simulink model "CL1CM2"  (R2024b)
settings: Solver=VariableStepAuto  StartTime=0.0  StopTime=10.0  RelTol=1e-3
settings Model: Creator=jeonghyun  LastModifiedBy=gluts

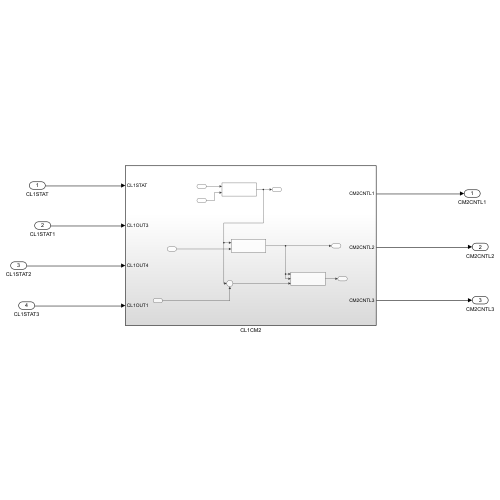
[thumbnail: Simulink's stored preview of the top-level diagram]
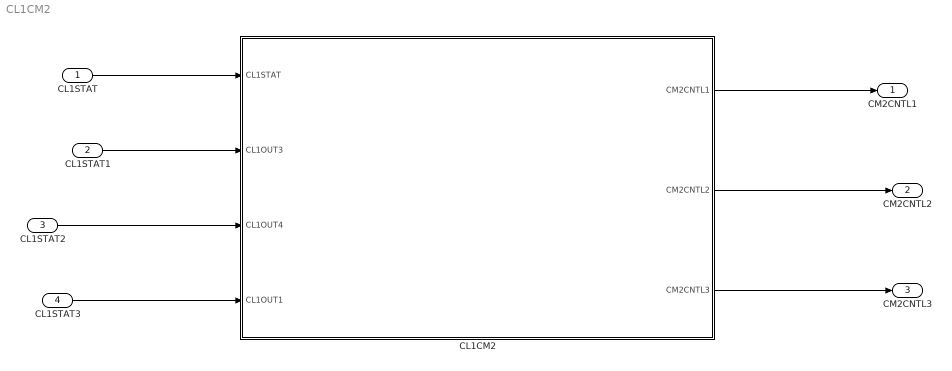
== system CL1CM2 ==
  CL1STAT : Inport
  CL1STAT1 : Inport  Port=2
  CL1STAT2 : Inport  Port=3
  CL1STAT3 : Inport  Port=4
  CL1CM2 : Subsystem
  CM2CNTL1 : Outport
  CM2CNTL2 : Outport  Port=2
  CM2CNTL3 : Outport  Port=3
  wires:
  CL1STAT/1 -> CL1CM2/1(CL1STAT)
  CL1STAT1/1 -> CL1CM2/2(CL1OUT3)
  CL1STAT2/1 -> CL1CM2/3(CL1OUT4)
  CL1STAT3/1 -> CL1CM2/4(CL1OUT1)
  CL1CM2/1(CM2CNTL1) -> CM2CNTL1/1
  CL1CM2/2(CM2CNTL2) -> CM2CNTL2/1
  CL1CM2/3(CM2CNTL3) -> CM2CNTL3/1

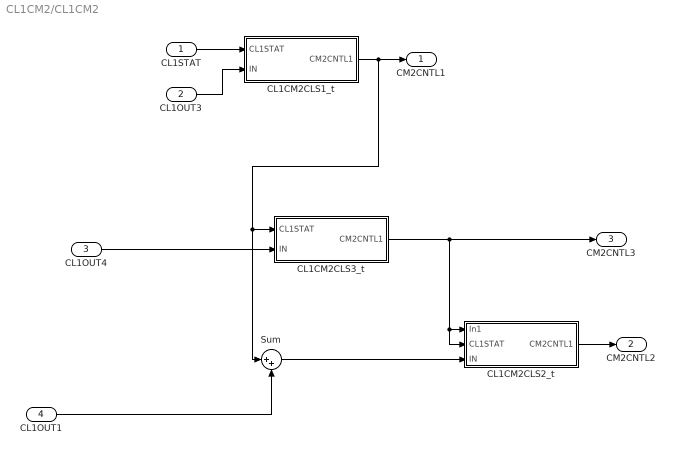
== system CL1CM2/CL1CM2 ==
  CL1STAT : Inport
  CL1OUT3 : Inport  Port=2
  CL1OUT4 : Inport  Port=3
  CL1OUT1 : Inport  Port=4
  CL1CM2CLS1_t : Subsystem
  CL1CM2CLS2_t : Subsystem
  CL1CM2CLS3_t : Subsystem
  Sum : Sum  Inputs=|++
  CM2CNTL1 : Outport
  CM2CNTL2 : Outport  Port=2
  CM2CNTL3 : Outport  Port=3
  wires:
  CL1STAT/1 -> CL1CM2CLS1_t/1(CL1STAT)
  CL1CM2CLS2_t/1(CM2CNTL1) -> CM2CNTL2/1
  CL1OUT3/1 -> CL1CM2CLS1_t/2(IN)
  CL1CM2CLS1_t/1(CM2CNTL1) -> CM2CNTL1/1, Sum/1, CL1CM2CLS3_t/1(CL1STAT)
  CL1OUT4/1 -> CL1CM2CLS3_t/2(IN)
  CL1CM2CLS3_t/1(CM2CNTL1) -> CL1CM2CLS2_t/1(In1), CL1CM2CLS2_t/2(CL1STAT), CM2CNTL3/1
  CL1OUT1/1 -> Sum/2
  Sum/1 -> CL1CM2CLS2_t/3(IN)

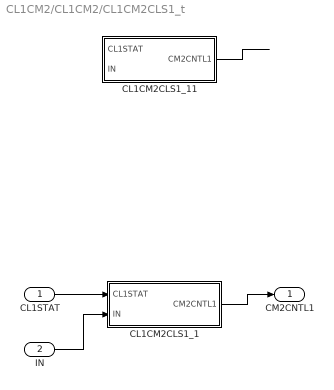
== system CL1CM2/CL1CM2/CL1CM2CLS1_t ==
  CL1STAT : Inport
  IN : Inport  Port=2
  CL1CM2CLS1_1 : Subsystem
  CL1CM2CLS1_11 : Subsystem
  CM2CNTL1 : Outport
  wires:
  CL1STAT/1 -> CL1CM2CLS1_1/1(CL1STAT)
  IN/1 -> CL1CM2CLS1_1/2(IN)
  CL1CM2CLS1_1/1(CM2CNTL1) -> CM2CNTL1/1
  CL1CM2CLS1_11/1(CM2CNTL1) -> ?
  ? -> CL1CM2CLS1_11/1(CL1STAT)
  ? -> CL1CM2CLS1_11/2(IN)

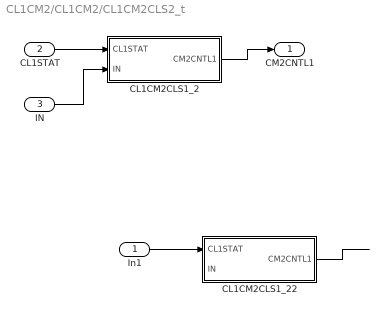
== system CL1CM2/CL1CM2/CL1CM2CLS2_t ==
  In1 : Inport
  CL1STAT : Inport  Port=2
  IN : Inport  Port=3
  CL1CM2CLS1_2 : Subsystem
  CL1CM2CLS1_22 : Subsystem
  CM2CNTL1 : Outport
  wires:
  CL1STAT/1 -> CL1CM2CLS1_2/1(CL1STAT)
  CL1CM2CLS1_2/1(CM2CNTL1) -> CM2CNTL1/1
  IN/1 -> CL1CM2CLS1_2/2(IN)
  In1/1 -> CL1CM2CLS1_22/1(CL1STAT)
  CL1CM2CLS1_22/1(CM2CNTL1) -> ?
  ? -> CL1CM2CLS1_22/2(IN)

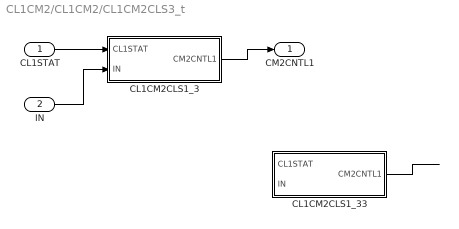
== system CL1CM2/CL1CM2/CL1CM2CLS3_t ==
  CL1STAT : Inport
  IN : Inport  Port=2
  CL1CM2CLS1_3 : Subsystem
  CL1CM2CLS1_33 : Subsystem
  CM2CNTL1 : Outport
  wires:
  CL1CM2CLS1_3/1(CM2CNTL1) -> CM2CNTL1/1
  CL1STAT/1 -> CL1CM2CLS1_3/1(CL1STAT)
  IN/1 -> CL1CM2CLS1_3/2(IN)
  ? -> CL1CM2CLS1_33/1(CL1STAT)
  CL1CM2CLS1_33/1(CM2CNTL1) -> ?
  ? -> CL1CM2CLS1_33/2(IN)

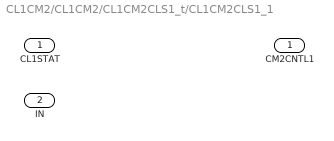
== system CL1CM2/CL1CM2/CL1CM2CLS1_t/CL1CM2CLS1_1 ==
  CL1STAT : Inport
  IN : Inport  Port=2
  CM2CNTL1 : Outport

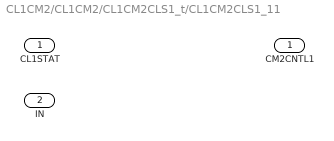
== system CL1CM2/CL1CM2/CL1CM2CLS1_t/CL1CM2CLS1_11 ==
  CL1STAT : Inport
  IN : Inport  Port=2
  CM2CNTL1 : Outport

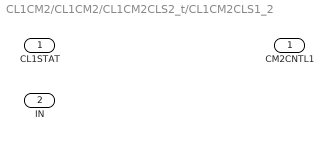
== system CL1CM2/CL1CM2/CL1CM2CLS2_t/CL1CM2CLS1_2 ==
  CL1STAT : Inport
  IN : Inport  Port=2
  CM2CNTL1 : Outport

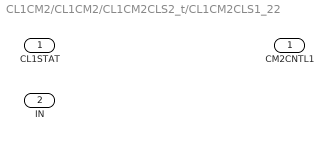
== system CL1CM2/CL1CM2/CL1CM2CLS2_t/CL1CM2CLS1_22 ==
  CL1STAT : Inport
  IN : Inport  Port=2
  CM2CNTL1 : Outport

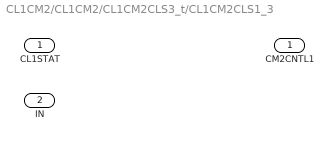
== system CL1CM2/CL1CM2/CL1CM2CLS3_t/CL1CM2CLS1_3 ==
  CL1STAT : Inport
  IN : Inport  Port=2
  CM2CNTL1 : Outport

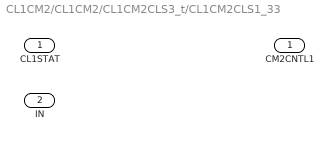
== system CL1CM2/CL1CM2/CL1CM2CLS3_t/CL1CM2CLS1_33 ==
  CL1STAT : Inport
  IN : Inport  Port=2
  CM2CNTL1 : Outport
